simulink model "InvertedPendulum"  (R2024b)
settings: Solver=VariableStepAuto  StartTime=0.0  StopTime=10.0  RelTol=1e-3
settings Model: Creator=kadir  LastModifiedBy=kadir

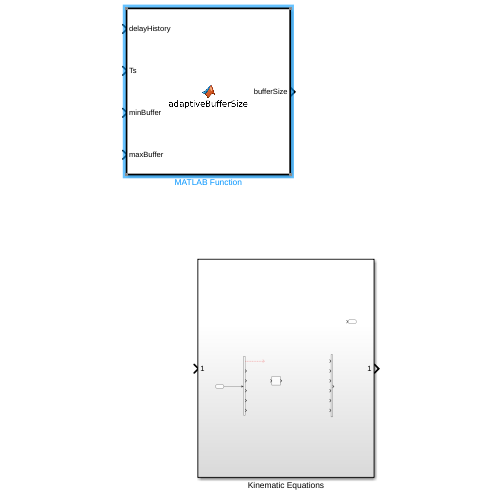
[thumbnail: Simulink's stored preview of the top-level diagram]
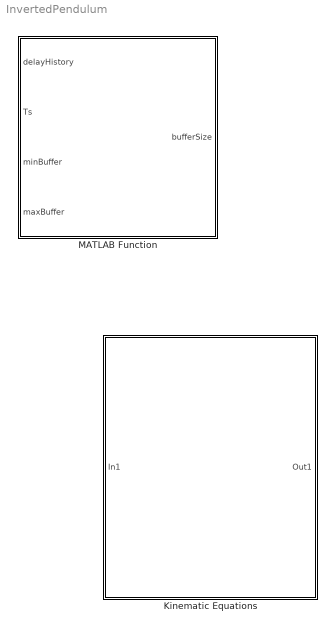
== system InvertedPendulum ==
  Kinematic Equations : Subsystem
  MATLAB Function : MATLAB Function  TreatAsAtomicUnit=on

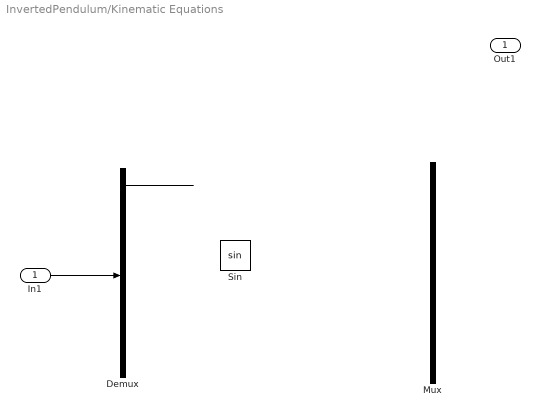
== system InvertedPendulum/Kinematic Equations ==
  In1 : Inport
  Demux : Demux  Outputs=6
  Mux : Mux  Inputs=6
  Sin : Trigonometry
  Out1 : Outport
  wires:
  In1/1 -> Demux/1
  Demux/1 -> ?

== matlab function InvertedPendulum/MATLAB Function ==
  data: delayHistory input; bufferSize output; Ts input; minBuffer input; maxBuffer input
function bufferSize = adaptiveBufferSize(delayHistory, Ts, minBuffer, maxBuffer)
    % Adaptive buffer size calculation for NCS
    % delayHistory: Gecikme ölçümlerinin vektörü (seconds)
    % Ts: Örnekleme Zamanı (saniye)
    % minBuffer, maxBuffer: Tampon bölgenin boyutu (paket sayısı)
    
    % Parametreler
    k1 = 0.8;   % Ortalama Gecikmenin Ağırlığı
    k2 = 1.2;   % Jitter Etkisinin Ağırlığı
    
    % Gecikme hesapları
    meanDelay = mean(delayHistory);
    stdDelay  = std(delayHistory);
    
    % Base buffer (at least 2 samples)
    baseSize = 2;
    
    % Yeni tampon boyutu hesaplama
    bufferSize = baseSize + k1 * (meanDelay / Ts) + k2 * (stdDelay / Ts);
    
    % Yuvarlama
    bufferSize = round(bufferSize);
    
    % Apply limits
    bufferSize = max(minBuffer, min(bufferSize, maxBuffer));
end
